simulink model "underwater_controller"  (R2026a)
settings: Solver=VariableStepAuto
InitFcn:
  | underwater_init
values from neighbouring files (symbols this model uses):
  A_face = [0.1; 0.1; 0.2]    [aerial_init.m]    (also in underwater_init.m = [W_box * H_box)
  Cd = [1.28; 1.28; 1.28]    [aerial_init.m]    (also in underwater_init.m = [1.2; 1.2; 1.5])
  F_buoyancy = rho_water * V_sub * g    (= 754.14375)    [underwater_init.m]
  g = 9.81    [aerial_init.m]    (also in underwater_init.m)
  gamma = deg2rad(gamma_deg)    [underwater_init.m]
  I_matrix_total = diag([Ixx + I_added(1), Iyy + I_added(2), Izz + I_added(3)])    [underwater_init.m]
  kQ_fwd = 1.0e-5    (= 1e-05)    [underwater_init.m]
  kQ_rev = 0.8e-5    (= 8e-06)    [underwater_init.m]
  kT_fwd = 5.0e-4    (= 0.0005)    [underwater_init.m]
  kT_rev = 4.0e-4    (= 0.0004)    [underwater_init.m]
  L_box = 0.50    (= 0.5)    [underwater_init.m]
  m = 25.0    (= 25)    [aerial_init.m]    (also in underwater_init.m)
  M_total = m + m_added    [underwater_init.m]
  rho_water = 1025.0    (= 1025)    [underwater_init.m]
  tau_m = 0.06    [aerial_init.m]    (also in underwater_init.m)
  tau_servo = 0.15    [underwater_init.m]
  W_box = 0.50    (= 0.5)    [underwater_init.m]
settings Model: Creator=banda  LastModifiedBy=banda

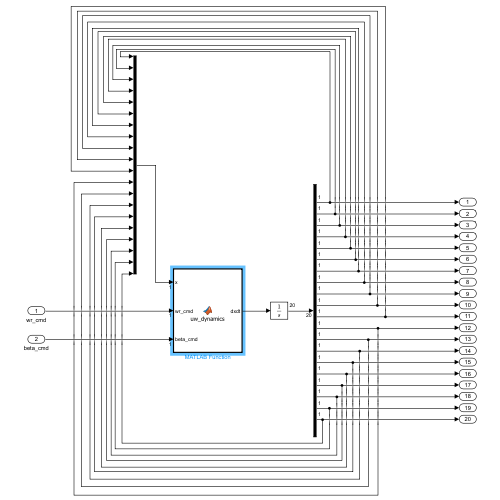
[thumbnail: Simulink's stored preview of the top-level diagram]
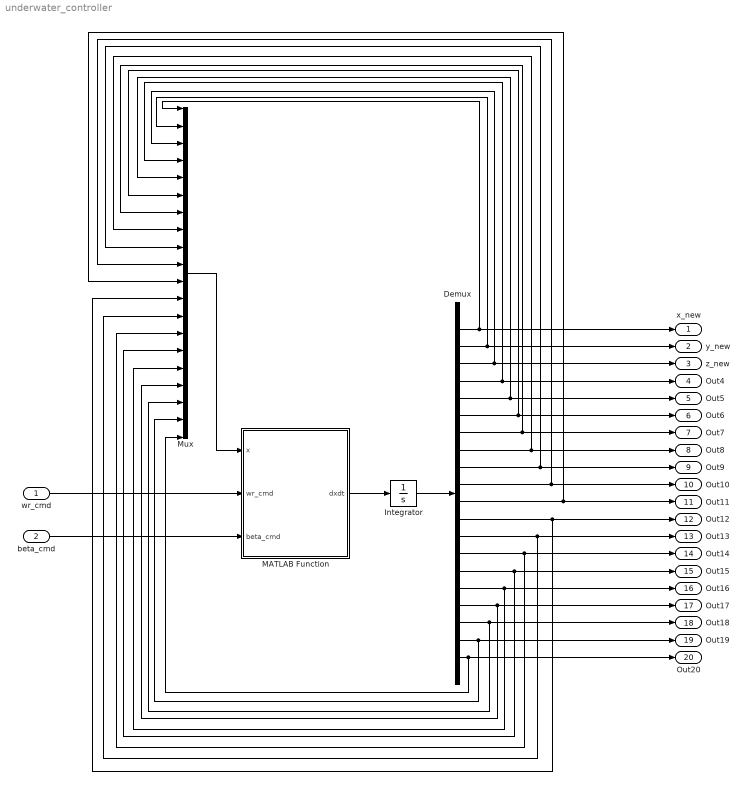
== system underwater_controller ==
  wr_cmd : Inport
  beta_cmd : Inport  Port=2
  Demux : Demux  Outputs=20
  Integrator : Integrator  InitialCondition=zeros(20,1)
  MATLAB Function : MATLAB Function  TreatAsAtomicUnit=on
  Mux : Mux  Inputs=20
  x_new : Outport
  y_new : Outport  Port=2
  z_new : Outport  Port=3
  Out4 : Outport  Port=4
  Out5 : Outport  Port=5
  Out6 : Outport  Port=6
  Out7 : Outport  Port=7
  Out8 : Outport  Port=8
  Out9 : Outport  Port=9
  Out10 : Outport  Port=10
  Out11 : Outport  Port=11
  Out12 : Outport  Port=12
  Out13 : Outport  Port=13
  Out14 : Outport  Port=14
  Out15 : Outport  Port=15
  Out16 : Outport  Port=16
  Out17 : Outport  Port=17
  Out18 : Outport  Port=18
  Out19 : Outport  Port=19
  Out20 : Outport  Port=20
  wires:
  MATLAB Function/1(dxdt) -> Integrator/1
  Integrator/1 -> Demux/1
  Demux/1 -> Mux/1, x_new/1
  Demux/2 -> y_new/1, Mux/2
  Demux/4 -> Out4/1, Mux/4
  Demux/3 -> z_new/1, Mux/3
  Demux/8 -> Mux/8, Out8/1
  Demux/12 -> Out12/1, Mux/12
  Demux/20 -> Out20/1, Mux/20
  Demux/5 -> Out5/1, Mux/5
  Demux/6 -> Out6/1, Mux/6
  Demux/7 -> Mux/7, Out7/1
  Demux/9 -> Out9/1, Mux/9
  Demux/10 -> Out10/1, Mux/10
  Demux/11 -> Mux/11, Out11/1
  Demux/13 -> Mux/13, Out13/1
  Demux/14 -> Out14/1, Mux/14
  Demux/15 -> Out15/1, Mux/15
  Demux/16 -> Out16/1, Mux/16
  Demux/17 -> Out17/1, Mux/17
  Demux/18 -> Out18/1, Mux/18
  Demux/19 -> Out19/1, Mux/19
  Mux/1 -> MATLAB Function/1(x)
  wr_cmd/1 -> MATLAB Function/2(wr_cmd)
  beta_cmd/1 -> MATLAB Function/3(beta_cmd)

== matlab function underwater_controller/MATLAB Function ==
  data: x input; dxdt output; wr_cmd input; beta_cmd input; kQ_rev parameter; kQ_fwd parameter; kT_rev parameter; kT_fwd parameter; tau_servo parameter; tau_m parameter; gamma parameter; W_box parameter; L_box parameter; A_face parameter; Cd parameter; F_buoyancy parameter; rho_water parameter; I_matrix_total parameter; M_total parameter; g parameter; m parameter
function dxdt = uw_dynamics(x, wr_cmd, beta_cmd, kQ_rev, kQ_fwd, kT_rev, kT_fwd, tau_servo, tau_m, gamma, W_box, L_box, A_face, Cd, F_buoyancy, rho_water, I_matrix_total, M_total, g, m)
% 20-State Underwater 6-DOF Dynamics 
% Bi-directional props on 180-degree servos with Added Mass/Inertia

% ---------------------------------------------------------------------
% 1. COLUMN ENFORCERS & STATE EXTRACTION
% ---------------------------------------------------------------------
x = x(:); wr_cmd = wr_cmd(:); beta_cmd = beta_cmd(:);
M_total = M_total(:); Cd = Cd(:); A_face = A_face(:);

% Extract states
pos   = x(1:3);                  % Inertial Position [x; y; z]
euler = x(4:6);                  % Attitude [phi; theta; psi]
vel   = x(7:9);                  % Inertial Velocity [xd; yd; zd]
wb    = x(10:12);                % Body Angular Rates [p; q; r]
wr    = x(13:16);                % Actual Prop Speeds (rad/s)
beta  = x(17:20);                % Actual Servo Angles (rad)

phi = euler(1); theta = euler(2); psi = euler(3);

% ---------------------------------------------------------------------
% 2. ACTUATOR GEOMETRY & THRUST MAPPING
% ---------------------------------------------------------------------
% Base direction vectors (gamma inward from walls) in XY plane
u1 = [ cos(gamma); -sin(gamma); 0]; % FL: Forward & Right
u2 = [ cos(gamma);  sin(gamma); 0]; % FR: Forward & Left
u3 = [-cos(gamma); -sin(gamma); 0]; % RL: Backward & Right
u4 = [-cos(gamma);  sin(gamma); 0]; % RR: Backward & Left
U_base = [u1, u2, u3, u4];

% Propeller positions in body frame (corners at COM height Z=0)
Lx = L_box/2; Ly = W_box/2;
r_props = [ Lx,  Ly, 0;    % FL
            Lx, -Ly, 0;    % FR
           -Lx,  Ly, 0;    % RL
           -Lx, -Ly, 0]';  % RR (3x4 matrix)

% Prop handedness [CCW, CW, CW, CCW] for standard configuration
h_dir = [1, -1, -1, 1];

F_prop_total = zeros(3,1);
tau_prop_total = zeros(3,1);

% Loop through all 4 vectoring thrusters
for i = 1:4
    % A. Bi-directional Thrust and Torque scaling
    if wr(i) >= 0
        T_i = kT_fwd * wr(i)^2;
        Q_i = kQ_fwd * wr(i)^2;
    else
        T_i = -kT_rev * wr(i)^2;
        Q_i = -kQ_rev * wr(i)^2;
    end
    
    % B. 3D Thrust Vector (v_i) defined by servo angle (beta)
    % beta=0 (horizontal), beta=pi/2 (vertical), beta=pi (horizontal reversed)
    v_i = cos(beta(i)) * U_base(:, i) + sin(beta(i)) * [0; 0; 1];
    
    % C. Resulting Force and Torques
    F_i = T_i * v_i;
    tau_thrust_i = cross(r_props(:, i), F_i);
    tau_rxn_i    = -h_dir(i) * Q_i * v_i; % Reaction opposes spin vector
    
    F_prop_total = F_prop_total + F_i;
    tau_prop_total = tau_prop_total + tau_thrust_i + tau_rxn_i;
end

% ---------------------------------------------------------------------
% 3. HYDRODYNAMICS & ADDED MASS (NEWTON-EULER)
% ---------------------------------------------------------------------
% Euler Rotation Matrix (Body to Inertial)
R = [ cos(psi)*cos(theta),  cos(psi)*sin(theta)*sin(phi) - sin(psi)*cos(phi),  cos(psi)*sin(theta)*cos(phi) + sin(psi)*sin(phi);
      sin(psi)*cos(theta),  sin(psi)*sin(theta)*sin(phi) + cos(psi)*cos(phi),  sin(psi)*sin(theta)*cos(phi) - cos(psi)*sin(phi);
     -sin(theta),           cos(theta)*sin(phi),                               cos(theta)*cos(phi) ];

% Calculate external forces IN THE BODY FRAME
v_body = R' * vel;
F_drag_body = -0.5 * rho_water * (Cd .* A_face) .* v_body .* abs(v_body);

F_gb_inertial = [0; 0; F_buoyancy - (m * g)];
F_gb_body = R' * F_gb_inertial;

% Sum all body forces
F_body_net = F_prop_total + F_drag_body + F_gb_body;

% Apply directional Added Mass (element-wise division in body frame)
accel_body = F_body_net ./ M_total;

% Rotate resulting acceleration back to inertial frame
pos_ddot = R * accel_body;

% Rotational dynamics using the pre-computed Effective Total Inertia
wb_dot = I_matrix_total \ (tau_prop_total - cross(wb, I_matrix_total * wb));

% ---------------------------------------------------------------------
% 4. KINEMATICS & ACTUATOR LAG
% ---------------------------------------------------------------------
euler_kin = [ 1,  sin(phi)*sin(theta)/cos(theta),  cos(phi)*sin(theta)/cos(theta);
              0,  cos(phi),                       -sin(phi);
              0,  sin(phi)/cos(theta),             cos(phi)/cos(theta) ];
euler_dot = euler_kin * wb;

% First-order lags for both motors and servos
wr_dot   = (wr_cmd - wr) / tau_m;
beta_dot = (beta_cmd - beta) / tau_servo;

% ---------------------------------------------------------------------
% 5. PACK DERIVATIVES (20 States)
% ---------------------------------------------------------------------
dxdt = [vel; euler_dot; pos_ddot; wb_dot; wr_dot; beta_dot];
end
